simulink model "UAM_Flight_control"  (R2024b)
settings: Solver=FixedStepAuto  StartTime=0.0  StopTime=inf  RelTol=1e-3  EnableMultiTasking=on
undefined symbols (not defined in the file): CityMission, control, controlParams, ControlSampleTime, Cruise_a, DiscIntNeverNeededParam, Earth, FixedWingMission, flightState, FSState, FWControlParams, FWTrimSpeed, HoverMission, params, position, R_WAYPOINTTRANSITION, TransitionMission, uavParam, Vt, w_trim, WGS84, zGround
libraries: slpidlib x56, simulink x32, uavalgslib x7, robotcorelib x2, simulink_extras x2, mspfiltlib x1, aerolibtransform2 x1
(part 11 of 13)

== matlab function UAM_Flight_control/Controller/Auto1/Fixed Wing Controller/Subsystem/Lateral Guidance Logic/MATLAB Function ==
  data: courseSP input; lacc output; course input; rollSP output; groundSpeed input; L1 input
function [lacc, rollSP] = fcn(courseSP, course, groundSpeed, L1)
eta = courseSP - course;

% wrap -pi to pi
eta = mod(eta, 2*pi);
if eta>pi
    eta = eta - 2*pi;
end

% cap eta to -pi/2 to pi/2
eta = min(eta, pi/2);
eta = max(eta, -pi/2);

lacc = 2*(groundSpeed^2)/L1*sin(eta);

rollSP = atan(lacc/9.81);

== matlab function UAM_Flight_control/Controller/Auto1/Fixed Wing Controller/Subsystem/Subsystem2/MATLAB Function ==
  data: phi input; y output; theta input
function y = fcn(phi,theta)

y=zeros(3,3);
y=[1 sin(phi)*tan(theta) cos(phi)*tan(theta); 0 cos(phi) -sin(phi); 0 sin(phi)/cos(theta) cos(phi)/cos(theta)];
end

== matlab function UAM_Flight_control/Controller/Emergency/FixedWing Controller/Subsystem/Attitude Controller/Pitch Roll Controller/Turn Coordinator/MATLAB Function ==
  data: rollSP input; rSP output; pitchSP input; airSpeed input
function rSP = fcn(rollSP, pitchSP, airSpeed)
    yawRateSP = tan(rollSP)*9.81/max(airSpeed,5);
    rSP = yawRateSP*cos(pitchSP)*cos(rollSP);
end

== matlab function UAM_Flight_control/Controller/Emergency/FixedWing Controller/Subsystem/Subsystem2/MATLAB Function ==
  data: phi input; y output; theta input
function y = fcn(phi,theta)

y=zeros(3,3);
y=[1 sin(phi)*tan(theta) cos(phi)*tan(theta); 0 cos(phi) -sin(phi); 0 sin(phi)/cos(theta) cos(phi)/cos(theta)];
end

== matlab function UAM_Flight_control/Controller/Manual/FixedWing Controller/Subsystem/Attitude Controller/Pitch Roll Controller/Turn Coordinator/MATLAB Function ==
  data: rollSP input; rSP output; pitchSP input; airSpeed input
function rSP = fcn(rollSP, pitchSP, airSpeed)
    yawRateSP = tan(rollSP)*9.81/max(airSpeed,5);
    rSP = yawRateSP*cos(pitchSP)*cos(rollSP);
end

== matlab function UAM_Flight_control/Controller/Manual/FixedWing Controller/Subsystem/Subsystem2/MATLAB Function ==
  data: phi input; y output; theta input
function y = fcn(phi,theta)

y=zeros(3,3);
y=[1 sin(phi)*tan(theta) cos(phi)*tan(theta); 0 cos(phi) -sin(phi); 0 sin(phi)/cos(theta) cos(phi)/cos(theta)];
end

== matlab function UAM_Flight_control/Controller/Manual/multicopter Controller/Attitude & Altitude controller/Derivative Gain/deadzone/MATLAB Function ==
  data: trigger input; yaw_sp output; euler_yaw input
function yaw_sp = yaw_hold(trigger, euler_yaw)
persistent last_yaw_sp

if isempty(last_yaw_sp)
    last_yaw_sp = 0;
end

if trigger == 1
    last_yaw_sp = euler_yaw;
end

yaw_sp = last_yaw_sp;

== matlab function UAM_Flight_control/Controller/Manual/Scheduler/Subsystem/Switch Case Action Subsystem/Desaturation ==
  data: m_in input; m_out output; mixMat input
%{
function m_out = desat_px4(m_in, mixMat)

% PX4-style desaturation (Stabilized, MC_AIRMODE=0, 튜닝용)

m = m_in(:);
[N, cols] = size(mixMat);
assert(numel(m)==N && cols==4, 'mixMat must be [Nm x 4]');

act_min = zeros(N,1);
act_max = ones(N,1);
MINIMUM_YAW_MARGIN = 0.15;

thrust_z = mixMat(:,1);
roll_vec = mixMat(:,2);
pitch_vec= mixMat(:,3);
yaw_vec  = mixMat(:,4);

% 1) thrust axis (thrust can only decrease)
m = desat_axis(m, thrust_z, act_min, act_max, true);

% 2) roll/pitch torques
m = desat_axis(m, roll_vec, act_min, act_max, false);
m = desat_axis(m, pitch_vec, act_min, act_max, false);

% 3) yaw with margin
act_max_yaw = act_max + (act_max - act_min) * MINIMUM_YAW_MARGIN;
m = desat_axis(m, yaw_vec, act_min, act_max_yaw, false);

% thrust again (only down)
m = desat_axis(m, thrust_z, act_min, act_max, true);

m_out = max(act_min, min(act_max, m));
end

function m = desat_axis(m, dir, act_min, act_max, thrust_only_down)
    k = compute_gain(dir, m, act_min, act_max);
    if ~(thrust_only_down && k > 0)
        m = m + k * dir;
    end

    k = 0.5 * compute_gain(dir, m, act_min, act_max);
    if ~(thrust_only_down && k > 0)
        m = m + k * dir;
    end
end

function k = compute_gain(dir, m, act_min, act_max)
    k_min = 0.0; 
    k_max = 0.0;

    for i = 1:numel(m)
        if abs(dir(i)) < 0.2
            continue;
        end

        if m(i) < act_min(i)
            ki = (act_min(i) - m(i)) / dir(i);
            k_min = min(k_min, ki);
            k_max = max(k_max, ki);
        end

        if m(i) > act_max(i)
            ki = (act_max(i) - m(i)) / dir(i);
            k_min = min(k_min, ki);
            k_max = max(k_max, ki);
        end
    end

    k = k_min + k_max;
end
%}

function m_out = desat_px4(m_in, mixMat)
% PX4-style desaturation (MC_AIRMODE = 1, Roll/Pitch airmode)

m = m_in(:);
[N, cols] = size(mixMat);
assert(numel(m)==N && cols==4, 'mixMat must be [Nm x 4]');

act_min = zeros(N,1);
act_max = ones(N,1);
MINIMUM_YAW_MARGIN = 0.15;

thrust_z = mixMat(:,1);
roll_vec  = mixMat(:,2); %#ok<NASGU>
pitch_vec = mixMat(:,3); %#ok<NASGU>
yaw_vec   = mixMat(:,4);

% 1) thrust axis (airmode: up/down 둘 다 허용)
m = desat_axis(m, thrust_z, act_min, act_max, false);

% 2) roll/pitch는 따로 줄이지 않음 (RP airmode: 자세 우선)

% 3) yaw with margin (mixYaw()와 동일 개념)
act_max_yaw = act_max + (act_max - act_min) * MINIMUM_YAW_MARGIN;
m = desat_axis(m, yaw_vec, act_min, act_max_yaw, false);

% 4) thrust again (only down, 0~1 안으로)
m = desat_axis(m, thrust_z, act_min, act_max, true);

m_out = max(act_min, min(act_max, m));
end

function m = desat_axis(m, dir, act_min, act_max, thrust_only_down)
    k = compute_gain(dir, m, act_min, act_max);
    if ~(thrust_only_down && k > 0)
        m = m + k * dir;
    end

    k = 0.5 * compute_gain(dir, m, act_min, act_max);
    if ~(thrust_only_down && k > 0)
        m = m + k * dir;
    end
end

function k = compute_gain(dir, m, act_min, act_max)
    k_min = 0.0;
    k_max = 0.0;

    for i = 1:numel(m)
        if abs(dir(i)) < 0.2
            continue;
        end

        if m(i) < act_min(i)
            ki = (act_min(i) - m(i)) / dir(i);
            k_min = min(k_min, ki);
            k_max = max(k_max, ki);
        end

        if m(i) > act_max(i)
            ki = (act_max(i) - m(i)) / dir(i);
            k_min = min(k_min, ki);
            k_max = max(k_max, ki);
        end
    end

    k = k_min + k_max;
end

== matlab function UAM_Flight_control/Controller/Manual/multicopter Controller/Attitude & Altitude controller/Derivative Gain/MATLAB Function ==
  data: x input; y output
function y = wrapToPi(x)
% x : angle error (rad)
% y : wrapped to [-pi, pi]
y = atan2(sin(x), cos(x));

== matlab function UAM_Flight_control/Controller/Manual/multicopter Controller/Atitude Control/MATLAB Function ==
  data: x input; y output
function y = wrapToPi(x)
% x : angle error (rad)
% y : wrapped to [-pi, pi]
y = atan2(sin(x), cos(x));

== matlab function UAM_Flight_control/Controller/Manual/multicopter Controller/Atitude Control/deadzone/MATLAB Function ==
  data: trigger input; yaw_sp output; euler_yaw input
function yaw_sp = yaw_hold(trigger, euler_yaw)
persistent last_yaw_sp

if isempty(last_yaw_sp)
    last_yaw_sp = 0;
end

if trigger == 1
    last_yaw_sp = euler_yaw;
end

yaw_sp = last_yaw_sp;

== matlab function UAM_Flight_control/Sensor/MATLAB Function ==
  data: pressure_kPa input; P0_Pa output; arm input; valid output
function [P0_Pa, valid] = latch_pressure_kPa(pressure_kPa, arm)
%#codegen
% Latch P0 at ARM rising edge (arm: 0 -> 1)

persistent p0_set p0_Pa last_arm
if isempty(p0_set)
    p0_set   = false;
    p0_Pa    = 0.0;
    last_arm = uint8(0);
end

P_Pa   = pressure_kPa * 1000.0;
arm_u8 = uint8(arm ~= 0);

% ---- Detect arm edge ----
arm_rising = (last_arm == 0) && (arm_u8 == 1);
arm_falling = (last_arm == 1) && (arm_u8 == 0);

% ---- ARM rising edge: latch P0 ----
if arm_rising
    if isfinite(P_Pa) && P_Pa > 0
        p0_Pa  = P_Pa;
        p0_set = true;
    else
        p0_Pa  = 0.0;
        p0_set = false;
    end
end

% ---- ARM falling edge: reset ----
if arm_falling
    p0_set = false;
    p0_Pa  = 0.0;
end

last_arm = arm_u8;

% ---- Outputs ----
P0_Pa = p0_Pa;
valid = p0_set;
end

== matlab function UAM_Flight_control/Sensor/Subsystem/MATLAB Function1 ==
  data: theta input; dq output
function dq = dq_from_theta(theta)
%#codegen
% theta: 3x1 = 0.5*(w-bg)*dt  (half-angle already applied)
% dq   : 4x1 quaternion increment [w;x;y;z]

a = sqrt(theta(1)^2 + theta(2)^2 + theta(3)^2);

if a < 1e-8
    % small-angle: sin(a)/a ≈ 1, cos(a) ≈ 1
    dq = [1.0;
          theta(1);
          theta(2);
          theta(3)];
else
    s = sin(a) / a;
    dq = [cos(a);
          theta(1)*s;
          theta(2)*s;
          theta(3)*s];
end
end

== matlab function UAM_Flight_control/Sensor/Subsystem/MATLAB Function2 ==
  data: q input; qout output; dq input
function qout = quat_mul(q, dq)
%#codegen
% qout = q ⊗ dq, both [w;x;y;z]
w1=q(1); x1=q(2); y1=q(3); z1=q(4);
w2=dq(1); x2=dq(2); y2=dq(3); z2=dq(4);

qout = [ w1*w2 - x1*x2 - y1*y2 - z1*z2;
         w1*x2 + x1*w2 + y1*z2 - z1*y2;
         w1*y2 - x1*z2 + y1*w2 + z1*x2;
         w1*z2 + x1*y2 - y1*x2 + z1*w2 ];
end

== matlab function UAM_Flight_control/Sensor/Subsystem/normalize ==
  data: q input; qn output
function qn = quat_norm(q)
%#codegen
n = sqrt(q(1)^2 + q(2)^2 + q(3)^2 + q(4)^2);
if n > 0
    qn = q / n;
else
    qn = [1;0;0;0];
end
end

== matlab function UAM_Flight_control/Sensor/MATLAB Function1 ==
  data: q input; R output
function R = quat_to_R_bn(q)
%#codegen
% q: [w; x; y; z] (unit quaternion)
% R: Body -> NED rotation matrix

w = q(1); x = q(2); y = q(3); z = q(4);

% Precompute products
ww = w*w; xx = x*x; yy = y*y; zz = z*z;

R = zeros(3,3);

R(1,1) = ww + xx - yy - zz;
R(1,2) = 2*(x*y - w*z);
R(1,3) = 2*(x*z + w*y);

R(2,1) = 2*(x*y + w*z);
R(2,2) = ww - xx + yy - zz;
R(2,3) = 2*(y*z - w*x);

R(3,1) = 2*(x*z - w*y);
R(3,2) = 2*(y*z + w*x);
R(3,3) = ww - xx - yy + zz;
end

== matlab function UAM_Flight_control/Sensor/MATLAB Function2 ==
  data: pressure_kPa input; z_baro output; P0_Pa input; P0_valid input
function z_baro = baro_z_from_pressure(pressure_kPa, P0_Pa, P0_valid)
%#codegen

% 입력 압력 (Pa)
P = pressure_kPa * 1000.0;

if ~P0_valid || P0_Pa <= 0
    z_baro = 0.0;
    return;
end

% ---- 고도 계산: P는 래치된 값 사용 ----
ratio = P / P0_Pa;
h_up  = 44330.0 * (1.0 - ratio.^0.1903); % Up(+), m
z_baro = -h_up;                         % NED Down(+)
end

== matlab function UAM_Flight_control/Sensor/MATLAB Function3 ==
  data: Pzz input; Pzz_n output; Pzv input; Pvv input; dt input; Qzz input; Qvv input; Pzv_n output; Pvv_n output
function [Pzz_n, Pzv_n, Pvv_n] = cov_predict(Pzz, Pzv, Pvv, dt, Qzz, Qvv)
%#codegen

Pzz_n = Pzz + 2*dt*Pzv + dt*dt*Pvv + Qzz;
Pzv_n = Pzv + dt*Pvv;
Pvv_n = Pvv + Qvv;

end

== matlab function UAM_Flight_control/Sensor/MATLAB Function4 ==
  data: gps_h_msl input; z_gps_ned output; ref_valid output
function [z_gps_ned, ref_valid] = latch_gps_z_firstvalid(gps_h_msl)
%#codegen
% gps_h_msl : GNSS absolute altitude (m, Up+). Some systems output 0 when invalid.
% z_gps_ned : relative altitude in NED Down(+) [m] (up -> negative)
% ref_valid : reference latched?

persistent ref_set h_ref last_z
if isempty(ref_set)
    ref_set = false;
    h_ref   = 0.0;
    last_z  = 0.0;
end

% ---- define validity check ----
% Treat non-finite or near-zero as invalid (tune threshold if your system can be near sea level).
is_valid = isfinite(gps_h_msl) && (abs(gps_h_msl) > 1.0);

% ---- latch reference on first valid sample ----
if ~ref_set && is_valid
    h_ref   = gps_h_msl;
    ref_set = true;
end

% ---- output ----
if ref_set && is_valid
    z_gps_ned = -(gps_h_msl - h_ref);
    last_z    = z_gps_ned;   % optional: hold last good output
    ref_valid = true;
else
    % If reference not ready or GPS temporarily invalid:
    z_gps_ned = last_z;      % hold last value (or 0.0 if you prefer)
    ref_valid = ref_set;     % true if we already latched ref at least once
end
end

== matlab function UAM_Flight_control/Sensor/MATLAB Function5 ==
  data: z_in input; z_lpf output; P0_valid input; valid output
function [z_lpf, valid] = lpf_z_baro(z_in, P0_valid)
%#codegen
% 1st-order discrete LPF:
%   y[k] = y[k-1] + alpha*(x[k] - y[k-1])
%
% Inputs:
%   z_in     : raw z_baro (m, NED Down +)
%   P0_valid : 0/1 (baro reference valid)
%
% Outputs:
%   z_lpf  : filtered z_baro
%   valid  : filtered output valid (same as P0_valid)

persistent y init
if isempty(init)
    y = 0.0;
    init = false;
end

% ---- Parameters (SET THESE) ----
Ts = 0.005;     % sample time [s] (200 Hz -> 0.005)
fc = 1.0;       % cutoff [Hz] (try 0.5~2.0)

% alpha = 1 - exp(-2*pi*fc*Ts)
alpha = 1.0 - exp(-2.0*pi*fc*Ts);

% ---- Valid handling ----
valid = (P0_valid ~= 0);

if ~valid || ~isfinite(z_in)
    % reset state when reference invalid
    y = 0.0;
    init = false;
    z_lpf = 0.0;
    return;
end

% ---- Initialize output to first input to avoid big transient ----
if ~init
    y = z_in;
    init = true;
    z_lpf = y;
    return;
end

% ---- LPF update ----
y = y + alpha*(z_in - y);
z_lpf = y;
end

== matlab function UAM_Flight_control/Controller/Manual/multicopter Controller/Altitude Control1/Normalization( -1 ~ 1)/MATLAB Function ==
  data: u input; y output; expo input
 function y = expo_curve(u, expo)                                                                                               
  % PX4 Exponential Curve                                                                                                        
  % u    : 입력 (-1 ~ 1 범위, Dead Zone 통과 후 정규화된 스틱 값)                                                                
  % expo : Expo 계수 (0 = 선형, 1 = 완전 큐빅, PX4 기본값 0.6)                                                                   
  % y    : 출력 (-1 ~ 1 범위)                                                                                                    
                                                                                                                                 
  y = sign(u) * (expo * abs(u)^3 + (1 - expo) * abs(u));                                                                         
                                                                                                                                 
  end

== matlab function UAM_Flight_control/Controller/Manual/multicopter Controller/Altitude Control1/MATLAB Function ==
  data: thrust_in input; vz input; az input; hover_est output; active input
  function hover_est = hover_thrust_lpf(thrust_in, vz, az, active)                                                  
      %#codegen                                            
      persistent hover_thrust                              
                                                           
      % Constants                                          
      HOVER_MIN = 0.2;                                     
      HOVER_MAX = 0.8;                                     
      SLEW_RATE = 0.0005;  % 200Hz 기준, 초당 0.1 변화     
      GRAVITY = 9.81;                                      
                                                           
      % Thresholds                                         
      VZ_LIM = 0.5;   % m/s                                
      AZ_LIM = 1.0;   % m/s²                               
                                                           
      if isempty(hover_thrust)                             
          hover_thrust = 0.5;                              
      end                                                  
                                                           
      hover_est = hover_thrust;                            
                                                           
      % 중력 제거                                          
      az_compensated = az + GRAVITY;                       
                                                           
      % 안정 조건 체크                                     
      is_stable = (abs(vz) < VZ_LIM) && (abs(az_compensated) < AZ_LIM);                          
                                                           
      if active && is_stable                               
          err = thrust_in - hover_thrust;                  
                                                           
          if err > SLEW_RATE                               
              hover_thrust = hover_thrust + SLEW_RATE;     
          elseif err < -SLEW_RATE                          
              hover_thrust = hover_thrust - SLEW_RATE;     
          else                                             
              hover_thrust = thrust_in;                    
          end                                              
                                                           
          hover_thrust = max(HOVER_MIN, min(HOVER_MAX, hover_thrust));                                          
      end                                                  
  end
